simulink model "CFunction"  (R2020a)
settings: Solver=FixedStepAuto  StartTime=0.0  StopTime=10.0  RelTol=1e-3
InitFcn:
  | %Motor1 = Epos4(1,0);
  | %Motor2 = Epos4(2,0);
model workspace (MAT data in the model file):
  NodeID = 1
  OperationMode = 0
  Ts = 0.001
CloseFcn:
  | delete(Motor1);
  | delete(Motor2);
settings Model: DataDictionary=MotorInfo.sldd  Creator=khoi  LastModifiedBy=khoi
settings RTWCC: GenCodeOnly=on

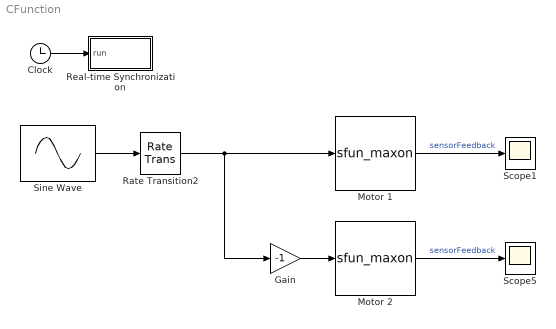
== system CFunction ==
  Clock : Clock
  Gain : Gain  Gain=-1
  Motor 1 : S-Function  FunctionName=sfun_maxon  Parameters=NodeID, DeltaT, OpMode  SFunctionDeploymentMode=off  EnableBusSupport=off  mask{NodeID=1, DeltaT=1e-3, OpMode=Cyclic synchronous velocity mode, P_cur=0, I_cur=0, P_pos=0, I_pos=0, D_pos=0, v_posGainFF=0, a_posGainFF=0, P_vel=0, I_vel=0, v_velGainFF=0, a_velGainFF=0, f_velCutoff=0}
      mask prompts: NodeID "Node ID"; DeltaT "Sample time (s)"; OpMode "Operation mode"; P_cur "P gain"; I_cur "I gain"; P_pos "P gain"; I_pos "I gain"; D_pos "D gain"; v_posGainFF "FF velocity gain"; a_posGainFF "FF acceleration gain"; P_vel "P gain"; I_vel "I gain"; v_velGainFF "Feed-forward velocity gain"; a_velGainFF "Feed-forward acceleration gain"; f_velCutoff "Filter cut-off frequency"
      mask TypeOptions OpMode: Cyclic synchronous current (torque) mode | Cyclic synchronous velocity mode | Cyclic synchronous position mode | Profile velocity mode | Profile position mode
      mask DialogControl DescGroupVar Prompt: Motor Parameters
      mask DialogControl Container6 Prompt: Motor
      mask DialogControl Container14 Prompt: Controller Parameters
      mask DialogControl DescTextVar_copy Prompt: This tab is experimental and does not implemented yet. Changing these parameters will not affect the motor performance.
      mask DialogControl Container15 Prompt: Current controller parameter set
      mask DialogControl Container15_copy Prompt: Position controller parameter set
      mask DialogControl Container15_copy_copy Prompt: Velocity controller parameter set
      mask Display:
      | disp('Maxon motor\nHIL');
      | % port_label('input', 1, 'inputSignal');
      | % port_label('output', 1, 'SENSR');
  Motor 2 : S-Function  FunctionName=sfun_maxon  Parameters=NodeID, DeltaT, OpMode  SFunctionDeploymentMode=off  EnableBusSupport=off  mask{NodeID=2, DeltaT=1e-3, OpMode=Cyclic synchronous velocity mode, P_cur=0, I_cur=0, P_pos=0, I_pos=0, D_pos=0, v_posGainFF=0, a_posGainFF=0, P_vel=0, I_vel=0, v_velGainFF=0, a_velGainFF=0, f_velCutoff=0}
      mask prompts: NodeID "Node ID"; DeltaT "Sample time"; OpMode "Operation mode"; P_cur "P gain"; I_cur "I gain"; P_pos "P gain"; I_pos "I gain"; D_pos "D gain"; v_posGainFF "FF velocity gain"; a_posGainFF "FF acceleration gain"; P_vel "P gain"; I_vel "I gain"; v_velGainFF "Feed-forward velocity gain"; a_velGainFF "Feed-forward acceleration gain"; f_velCutoff "Filter cut-off frequency"
      mask TypeOptions OpMode: Cyclic synchronous current (torque) mode | Cyclic synchronous velocity mode | Cyclic synchronous position mode | Profile velocity mode | Profile position mode
      mask DialogControl DescGroupVar Prompt: Motor Parameters
      mask DialogControl Container6 Prompt: Motor
      mask DialogControl Container14 Prompt: Controller Parameters
      mask DialogControl DescTextVar_copy Prompt: This tab is experimental and does not implemented yet. Changing these parameters will not affect the motor performance.
      mask DialogControl Container15 Prompt: Current controller parameter set
      mask DialogControl Container15_copy Prompt: Position controller parameter set
      mask DialogControl Container15_copy_copy Prompt: Velocity controller parameter set
      mask Display:
      | disp('Maxon motor\nHIL');
      | % port_label('input', 1, 'inputSignal');
      | % port_label('output', 1, 'SENSR');
  Rate Transition2 : RateTransition
  Real-time Synchronization : Subsystem
  Scope1 : Scope
  Scope5 : Scope
  Sine Wave : Sin  Amplitude=2000  SampleTime=0
  wires:
  Clock/1 -> Real-time Synchronization/1(run)
  Motor 2/1 -> Scope5/1  "sensorFeedback"
  Rate Transition2/1 -> Gain/1, Motor 1/1
  Sine Wave/1 -> Rate Transition2/1
  Gain/1 -> Motor 2/1
  Motor 1/1 -> Scope1/1  "sensorFeedback"

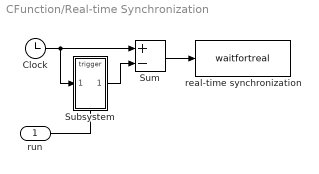
== system CFunction/Real-time Synchronization ==
  run : Inport
  Clock : Clock
  Subsystem : Subsystem  TreatAsAtomicUnit=on
  Sum : Sum  Inputs=+-  InputSameDT=on  SaturateOnIntegerOverflow=on  OutDataTypeStr=Inherit: Same as first input
  real-time synchronization : MATLABFcn  MATLABFcn=waitfortreal  OutputDimensions=0
  wires:
  Clock/1 -> Subsystem/1(In), Sum/1
  Subsystem/1(Out) -> Sum/2
  Sum/1 -> real-time synchronization/1
  run/1 -> Subsystem/Trigger

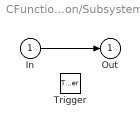
== system CFunction/Real-time Synchronization/Subsystem ==
  In : Inport
  Trigger : TriggerPort  VariantControl=(inherit)
  Out : Outport  InitialOutput=0
  wires:
  In/1 -> Out/1
